simulink model "controller_stateflow_2021a"  (R2021a)
settings: Solver=FixedStepAuto  StartTime=0.0  StopTime=inf  FixedStep=0.05  RelTol=1e-3
PreLoadFcn:
  | rosinit();
model workspace (MAT data in the model file):
  SL_ROS_VariableLengthArrays_MaxSizes.CommonInfo.ArrayTruncateAction = 'EmitWarning'
  SL_ROS_VariableLengthArrays_MaxSizes.MsgTypeMap = containers.Map
  SL_ROS_VariableLengthArrays_MaxSizes.MsgTypeMap.serialization.keys = {'gazebo_msgs/LinkStates', 'trajectory_msgs/JointTrajectory', 'trajectory_msgs/JointTrajectoryPoint'}
  SL_ROS_VariableLengthArrays_MaxSizes.MsgTypeMap.serialization.values{1}(1).PropertyName = 'Name'
  SL_ROS_VariableLengthArrays_MaxSizes.MsgTypeMap.serialization.values{1}(1).DataType = 'std_msgs/String'
  SL_ROS_VariableLengthArrays_MaxSizes.MsgTypeMap.serialization.values{1}(1).MaxLength = 100
  SL_ROS_VariableLengthArrays_MaxSizes.MsgTypeMap.serialization.values{1}(2).PropertyName = 'Pose'
  SL_ROS_VariableLengthArrays_MaxSizes.MsgTypeMap.serialization.values{1}(2).DataType = 'geometry_msgs/Pose'
  SL_ROS_VariableLengthArrays_MaxSizes.MsgTypeMap.serialization.values{1}(2).MaxLength = 100
  SL_ROS_VariableLengthArrays_MaxSizes.MsgTypeMap.serialization.values{1}(3).PropertyName = 'Twist'
  SL_ROS_VariableLengthArrays_MaxSizes.MsgTypeMap.serialization.values{1}(3).DataType = 'geometry_msgs/Twist'
  SL_ROS_VariableLengthArrays_MaxSizes.MsgTypeMap.serialization.values{1}(3).MaxLength = 100
  SL_ROS_VariableLengthArrays_MaxSizes.MsgTypeMap.serialization.values{2}(1).PropertyName = 'JointNames'
  SL_ROS_VariableLengthArrays_MaxSizes.MsgTypeMap.serialization.values{2}(1).DataType = 'std_msgs/String'
  SL_ROS_VariableLengthArrays_MaxSizes.MsgTypeMap.serialization.values{2}(1).MaxLength = 16
  SL_ROS_VariableLengthArrays_MaxSizes.MsgTypeMap.serialization.values{2}(2).PropertyName = 'Points'
  SL_ROS_VariableLengthArrays_MaxSizes.MsgTypeMap.serialization.values{2}(2).DataType = 'trajectory_msgs/JointTrajectoryPoint'
  SL_ROS_VariableLengthArrays_MaxSizes.MsgTypeMap.serialization.values{2}(2).MaxLength = 1
  SL_ROS_VariableLengthArrays_MaxSizes.MsgTypeMap.serialization.values{3}(1).PropertyName = 'Accelerations'
  SL_ROS_VariableLengthArrays_MaxSizes.MsgTypeMap.serialization.values{3}(1).DataType = 'double'
  SL_ROS_VariableLengthArrays_MaxSizes.MsgTypeMap.serialization.values{3}(1).MaxLength = 128
  SL_ROS_VariableLengthArrays_MaxSizes.MsgTypeMap.serialization.values{3}(2).PropertyName = 'Effort'
  SL_ROS_VariableLengthArrays_MaxSizes.MsgTypeMap.serialization.values{3}(2).DataType = 'double'
  SL_ROS_VariableLengthArrays_MaxSizes.MsgTypeMap.serialization.values{3}(2).MaxLength = 128
  SL_ROS_VariableLengthArrays_MaxSizes.MsgTypeMap.serialization.values{3}(3).PropertyName = 'Positions'
  SL_ROS_VariableLengthArrays_MaxSizes.MsgTypeMap.serialization.values{3}(3).DataType = 'double'
  SL_ROS_VariableLengthArrays_MaxSizes.MsgTypeMap.serialization.values{3}(3).MaxLength = 7
  SL_ROS_VariableLengthArrays_MaxSizes.MsgTypeMap.serialization.values{3}(4).PropertyName = 'Velocities'
  SL_ROS_VariableLengthArrays_MaxSizes.MsgTypeMap.serialization.values{3}(4).DataType = 'double'
  SL_ROS_VariableLengthArrays_MaxSizes.MsgTypeMap.serialization.values{3}(4).MaxLength = 128
  SL_ROS_VariableLengthArrays_MaxSizes.MsgTypeMap.serialization.uniformity = 0
  SL_ROS_VariableLengthArrays_MaxSizes.MsgTypeMap.serialization.keyType = 'char'
  SL_ROS_VariableLengthArrays_MaxSizes.MsgTypeMap.serialization.valueType = 'any'
  pitch = -10
  restart = 0
values from neighbouring files (symbols this model uses):
  Pose = distance*inv(toPandatf)*Pose_d0    [inverseContoller3.m]    (also in inverseContoller4.m = distance*inv(toUR10etf)*Point_d0; inverseContoller_dual.m = inv(toUR10etf)*Point_d0; inverseContoller_dual2.m = inv(toUR10etf)*Point_d0)
undefined symbols (not defined in the file or in its folder): StartTime
libraries: robotlib x19, robotmaniplib x5, robotcorelib x3, robotgazebolib x1
(part 1 of 2)
settings Model: Creator=marco  LastModifiedBy=marco
settings OptimizationCC: EnhancedBackFolding=on  PassReuseOutputArgsAs=Individual arguments  ZeroExternalMemoryAtStartup=off  ZeroInternalMemoryAtStartup=off  MaxStackSize=64  OptimizeBlockOrder=speed  DifferentSizesBufferReuse=on  OptimizationCustomize=off  EfficientTunableParamExpr=on
settings DebuggingCC: ParameterTunabilityLossMsg=error  UnconnectedInputMsg=none  UnconnectedOutputMsg=none  UnconnectedLineMsg=none
settings HardwareCC: ProdBitPerPointer=32  ProdBitPerSizeT=32  ProdBitPerPtrDiffT=32  ProdLargestAtomicFloat=None  ProdIntDivRoundTo=Undefined  ProdEndianess=Unspecified  ProdWordSize=32  ProdHWDeviceType=Generic->Unspecified (assume 32-bit Generic)
settings ModelReferenceCC: EnableRefExpFcnMdlSchedulingChecks=off
settings SFSimCC: MATLABDynamicMemAlloc=off
settings RTWCC: SystemTargetFile=ert.tlc  HardwareBoard=Robot Operating System (ROS)  TLCOptions="-aInlineSetEventsForThisBaseRateFcn=TLC_FALSE -aSuppressMultiTaskScheduler=TLC_FALSE  -aRateBasedStepFcn=0"  TemplateMakefile=ert_default_tmf  Toolchain=Catkin  TargetLang=C++  DLArmComputeVersion=20.02.1
settings CodeAppCC: ForceParamTrailComments=on  IgnoreCustomStorageClasses=off  OperatorAnnotations=on  SimulinkDataObjDesc=on  SFDataObjDesc=on  InsertBlockDesc=on

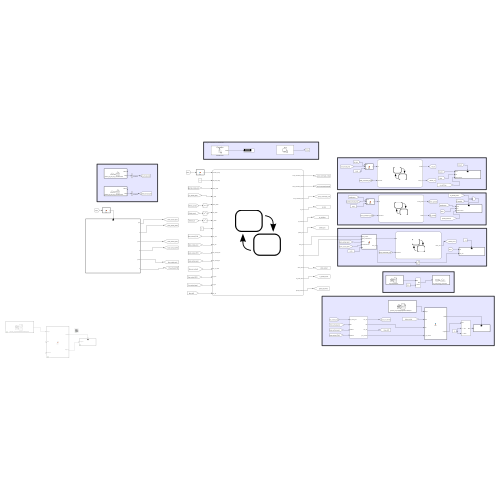
[thumbnail: Simulink's stored preview of the top-level diagram]
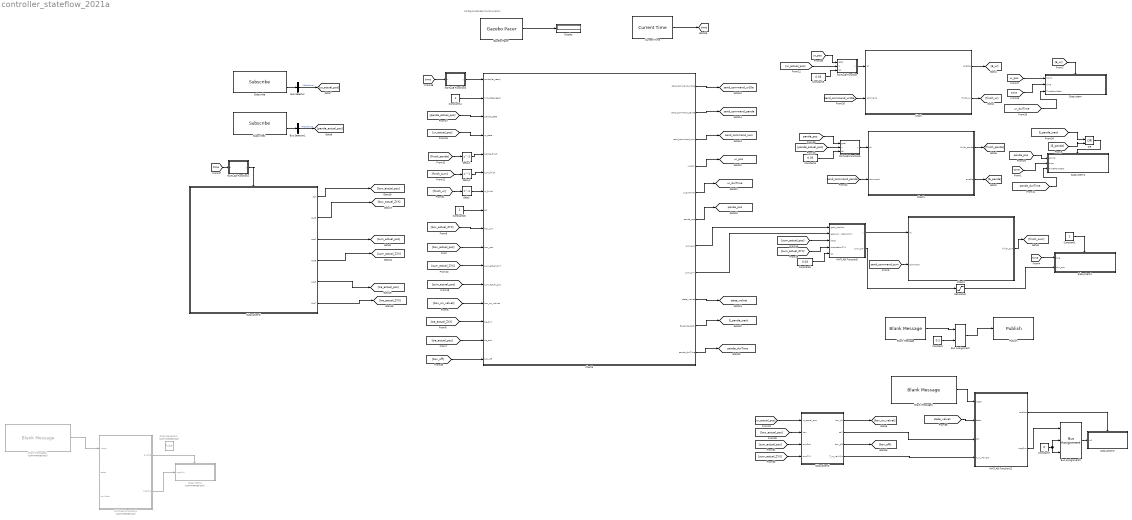
== system controller_stateflow_2021a ==
  note: Configure Gazebo Co-Simulation
  Blank Message : robotlib/Blank Message  messageClass=Message  entityType=std_msgs/Float64  messageType=std_msgs/Float64  SampleTime=inf  legacyBusStruct=off
  Blank Message1 : robotlib/Blank Message  messageClass=Service Request  entityType=gazebo_msgs/ApplyBodyWrench  messageType=gazebo_msgs/ApplyBodyWrenchRequest  SampleTime=-1  legacyBusStruct=off
  Blank Message2 : robotlib/Blank Message  Commented=on  messageClass=Service Request  entityType=gazebo_msgs/SetModelState  messageType=gazebo_msgs/SetModelStateRequest  SampleTime=-1  legacyBusStruct=off
  Bus Assignment : BusAssignment  AssignedSignals=Data
  Bus Assignment2 : BusAssignment  AssignedSignals=StartTime.Sec,StartTime.Nsec
  Bus Selector : BusSelector  OutputSignals=Actual.Positions
  Bus Selector1 : BusSelector  OutputSignals=Actual.Positions
  Chart : Stateflow chart  TreatAsAtomicUnit=on
  Chart1 : Stateflow chart  TreatAsAtomicUnit=on
  Chart2 : Stateflow chart  TreatAsAtomicUnit=on
  Chart3 : Stateflow chart  TreatAsAtomicUnit=on
  Constant : Constant  Value=0.2
  Constant1 : Constant
  Constant11 : Constant
  Constant20 : Constant
  Constant3 : Constant  Value=0.03
  Constant4 : Constant  Value=0.03
  Constant6 : Constant  Value=0.03
  Constant7 : Constant  Value=0
  Current Time : robotlib/Current Time  OutputFormat=bus  SampleTime=-1  ModelName=controller_stateflow
  Delay : Delay  DelayLength=1  InitialCondition=0
  Delay1 : Delay  DelayLength=1  InitialCondition=0
  Delay2 : Delay  DelayLength=1  InitialCondition=0
  Display : Display
  Gazebo Pacer : robotgazebolib/Gazebo Pacer  ResetBehavior=Reset Gazebo simulation time  SampleTime=0.05
  MATLAB Function : MATLAB Function  TreatAsAtomicUnit=on
  MATLAB Function1 : MATLAB Function  TreatAsAtomicUnit=on
  MATLAB Function12 : MATLAB Function  TreatAsAtomicUnit=on
  MATLAB Function14 : MATLAB Function  Commented=on  TreatAsAtomicUnit=on
  MATLAB Function2 : MATLAB Function  TreatAsAtomicUnit=on
  MATLAB Function3 : MATLAB Function  TreatAsAtomicUnit=on
  MATLAB Function5 : MATLAB Function  TreatAsAtomicUnit=on
  OR : Logic  Operator=OR  IconShape=distinctive  AllPortsSameDT=off  OutDataTypeStr=boolean
  Publish : robotlib/Publish  topicSource=Select from ROS network  topic=/right_hand_v1s/synergy_command  messageType=std_msgs/Float64  legacyBusStruct=off  messageQueueLength=1
  Pulse Generator : DiscretePulseGenerator  Commented=on  PulseType=Time based  Period=10  PulseWidth=0.1
  Saturation : Saturate  UpperLimit=0.2  LowerLimit=-0.2
  Subscribe : robotlib/Subscribe  topicSource=Select from ROS network  topic=/ur10e_eff_joint_traj_controller/state  messageType=control_msgs/JointTrajectoryControllerState  SampleTime=-1  legacyBusStruct=off  messageQueueLength=1
  Subscribe1 : robotlib/Subscribe  topicSource=Select from ROS network  topic=/panda_eff_joint_traj_controller/state  messageType=control_msgs/JointTrajectoryControllerState  SampleTime=-1  legacyBusStruct=off  messageQueueLength=1
  Subsystem : Subsystem
  Subsystem1 : Subsystem
  Subsystem2 : Subsystem
  Subsystem3 : Subsystem
  Subsystem4 : Subsystem  Commented=on
  Subsystem5 : Subsystem
  Subsystem6 : Subsystem
  tag scope: E_panda_track=global, panda_durTime=global, panda_pos=global, send_command_panda=global, send_command_sum=global, send_command_ur10e=global, state_velvet=global, time=global, ur_durTime=global, ur_pos=global
  wires:
  [time] -> Subsystem1/2(time)
  [E_ur] -> Subsystem/Enable
  Chart/1(enable) -> [E_ur]
  Subscribe/2 -> Bus Selector/1
  Constant3/1 -> MATLAB Function/3(tol)
  MATLAB Function/1(y) -> Chart/1(ok)
  MATLAB Function3/1(y) -> Chart1/1(ok)
  Constant4/1 -> MATLAB Function3/3(tol)
  Subscribe1/2 -> Bus Selector1/1
  Chart1/2(enable) -> [E_panda]
  [E_panda] -> OR/2
  [panda_pos] -> Subsystem1/1(points)
  Constant6/1 -> MATLAB Function5/5(tol)
  MATLAB Function5/1(y) -> Chart2/1(ok)
  MATLAB Function5/2(sum_cntr) -> Saturation/1
  Constant1/1 -> Subsystem2/Enable
  Chart/2(finish_ur) -> [finish_ur]
  Chart1/1(finish_panda) -> [finish_panda]
  Saturation/1 -> Subsystem2/2(sum_cntr)
  MATLAB Function1/1(y) -> Subsystem6/Enable
  Constant11/1 -> Chart3/2(link_state_ready)
  Bus Selector/1 -> [ur_actual_pos]  "<Positions>"
  Bus Selector1/1 -> [panda_actual_pos]  "<Positions>"
  [ur_actual_pos] -> MATLAB Function/2(u)
  [sum_actual_ZYX] -> MATLAB Function5/4(orientationZYX)
  [panda_actual_pos] -> MATLAB Function3/2(u)
  [panda_actual_pos] -> Chart3/3(panda_state)
  [ur_actual_pos] -> Chart3/4(ur_state)
  [finish_sum] -> Delay2/1
  [finish_ur] -> Delay/1
  Chart3/7(sum_pos) -> MATLAB Function5/1(goal_position)
  Delay/1 -> Chart3/7(ur_finish)
  Constant20/1 -> Chart3/8(go)
  [time] -> Subsystem/2(time)
  Chart3/1(send_command_ur10e) -> [send_command_ur10e]
  [send_command_ur10e] -> Chart/2(command)
  [ur_pos] -> Subsystem/1(Point)
  [ur_pos] -> MATLAB Function/1(goal)
  Chart3/3(send_command_sum) -> [send_command_sum]
  Chart3/2(send_command_panda) -> [send_command_panda]
  Chart3/4(ur_pos) -> [ur_pos]
  Chart3/6(panda_pos) -> [panda_pos]
  [send_command_panda] -> Chart1/2(command)
  [panda_pos] -> MATLAB Function3/1(goal)
  [finish_panda] -> Delay1/1
  Delay1/1 -> Chart3/5(panda_finish)
  [time] -> Subsystem2/1(time)
  [send_command_sum] -> Chart2/2(command)
  Chart2/1(finish_sum) -> [finish_sum]
  Delay2/1 -> Chart3/6(sum_finish)
  [box_actual_ZYX] -> Chart3/9(box_ZYX)
  Chart3/8(sum_ZYX) -> MATLAB Function5/2(goal_orientationZYX)
  [box_actual_pos] -> Chart3/10(box_pos)
  [sum_actual_pos] -> MATLAB Function5/3(pose)
  [sum_actual_ZYX] -> Chart3/11(sum_actual_ZYX)
  [sum_actual_pos] -> Chart3/12(sum_actual_pos)
  [box_on_velvet] -> Chart3/13(box_on_velvet)
  Bus Assignment/1 -> Publish/1
  Blank Message/1 -> Bus Assignment/1
  Constant/1 -> Bus Assignment/2
  [tra_actual_pos] -> Chart3/15(tra_pos)
  [tra_actual_ZYX] -> Chart3/14(tra_ZYX)
  OR/1 -> Subsystem1/Enable
  [panda_durTime] -> Subsystem1/3(TimeFromStart)
  Chart3/5(ur_durTime) -> [ur_durTime]
  [ur_durTime] -> Subsystem/3(TimeFromStart)
  Chart3/11(panda_durTime) -> [panda_durTime]
  MATLAB Function12/1(enable) -> Subsystem3/Enable
  Blank Message1/1 -> MATLAB Function12/1(msgIn)
  Bus Assignment2/1 -> Subsystem3/1(In1)
  Constant7/1 -> Bus Assignment2/3, Bus Assignment2/2
  MATLAB Function12/2(msgOut) -> Bus Assignment2/1
  Chart3/10(E_panda_track) -> [E_panda_track]
  [E_panda_track] -> OR/1
  Blank Message2/1 -> MATLAB Function14/1(msgIn)
  MATLAB Function14/2(msgOut) -> Subsystem4/1(msgOut)
  MATLAB Function14/1(enable) -> Subsystem4/Enable
  [box_off] -> Chart3/16(box_off)
  Chart3/9(state_velvet) -> [state_velvet]
  [state_velvet] -> MATLAB Function12/2(state)
  [ur_actual_pos] -> Subsystem5/1(ur_actual_pos)
  [box_actual_pos] -> Subsystem5/2(box)
  [sum_actual_pos] -> Subsystem5/3(sumPos)
  [sum_actual_ZYX] -> Subsystem5/4(sumZYX)
  Subsystem5/1(box_ok) -> [box_on_velvet]
  Subsystem5/2(coll) -> MATLAB Function12/3(coll)
  Subsystem5/3(box_off) -> [box_off]
  Subsystem5/4(T_ur_velvCnt) -> MATLAB Function12/4(T_ur_velvCnt)
  Gazebo Pacer/1 -> Display/1
  Subsystem6/1(pos) -> [box_actual_pos]
  Subsystem6/2(Out2) -> [box_actual_ZYX]
  Subsystem6/3(pos1) -> [sum_actual_pos]
  Subsystem6/4(Out5) -> [sum_actual_ZYX]
  Subsystem6/5(pos2) -> [tra_actual_pos]
  Subsystem6/6(Out7) -> [tra_actual_ZYX]
  [time] -> MATLAB Function1/1(u)
  Current Time/1 -> [time]
  [time] -> MATLAB Function2/1(u)
  MATLAB Function2/1(y) -> Chart3/1(controller_ready)

== system controller_stateflow_2021a/Chart3/THE_END ==
  go : Inport
  Action Port : ActionPort
      settings: CopyFcn=Stateflow.SLINSF.SimulinkMan.removeBlockPreDeleteFcn  PreDeleteFcn=Stateflow.SLINSF.SimulinkMan.unsafePredeleteFcn
  Stop Simulation : Stop
  wires:
  go/1 -> Stop Simulation/1

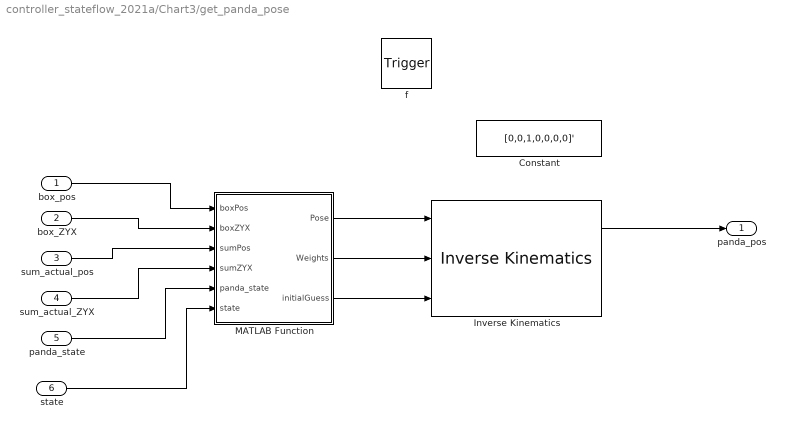
== system controller_stateflow_2021a/Chart3/get_panda_pose ==
  box_pos : Inport  OutDataTypeStr=double  PortDimensions=[3,1]
  box_ZYX : Inport  Port=2  OutDataTypeStr=double  PortDimensions=[3,1]
  sum_actual_pos : Inport  Port=3  OutDataTypeStr=double  PortDimensions=[3,1]
  sum_actual_ZYX : Inport  Port=4  OutDataTypeStr=double  PortDimensions=[3,1]
  panda_state : Inport  Port=5  OutDataTypeStr=double  PortDimensions=[7,1]
  state : Inport  Port=6  OutDataTypeStr=double  PortDimensions=1
  f : TriggerPort  TriggerType=function-call  VariantControl=(inherit)
      settings: CopyFcn=Stateflow.SLINSF.SimulinkMan.removeBlockPreDeleteFcn  PreDeleteFcn=Stateflow.SLINSF.SimulinkMan.unsafePredeleteFcn
  Constant : Constant  Value=[0,0,1,0,0,0,0]'
  Inverse Kinematics : robotmaniplib/Inverse Kinematics  RigidBodyTree=franka  EndEffector=hand_link  ShowInfo=on  SolverName=BFGS Gradient Projection  EnforceJointLimits=on  MaxIterations=1500  MaxTime=10  GradientTolerance=1e-7  SolutionTolerance=1e-6  StepTolerance=1e-14  ErrorChangeTolerance=1e-12  UseErrorDamping=on  DampingBias=0.0025  SimulateUsing=Interpreted execution
  MATLAB Function : MATLAB Function  TreatAsAtomicUnit=on
  panda_pos : Outport
  wires:
  panda_state/1 -> MATLAB Function/5(panda_state)
  box_pos/1 -> MATLAB Function/1(boxPos)
  box_ZYX/1 -> MATLAB Function/2(boxZYX)
  sum_actual_pos/1 -> MATLAB Function/3(sumPos)
  sum_actual_ZYX/1 -> MATLAB Function/4(sumZYX)
  MATLAB Function/1(Pose) -> Inverse Kinematics/1
  MATLAB Function/2(Weights) -> Inverse Kinematics/2
  MATLAB Function/3(initialGuess) -> Inverse Kinematics/3
  Inverse Kinematics/1 -> panda_pos/1
  state/1 -> MATLAB Function/6(state)

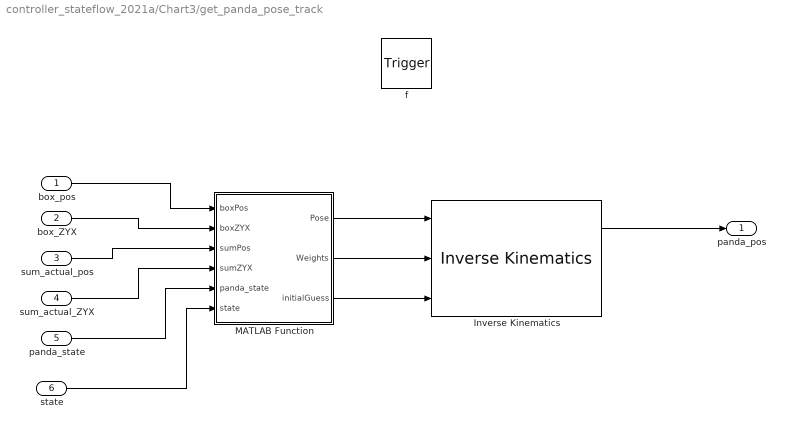
== system controller_stateflow_2021a/Chart3/get_panda_pose_track ==
  box_pos : Inport  OutDataTypeStr=double  PortDimensions=[3,1]
  box_ZYX : Inport  Port=2  OutDataTypeStr=double  PortDimensions=[3,1]
  sum_actual_pos : Inport  Port=3  OutDataTypeStr=double  PortDimensions=[3,1]
  sum_actual_ZYX : Inport  Port=4  OutDataTypeStr=double  PortDimensions=[3,1]
  panda_state : Inport  Port=5  OutDataTypeStr=double  PortDimensions=[7,1]
  state : Inport  Port=6  OutDataTypeStr=double  PortDimensions=1
  f : TriggerPort  TriggerType=function-call  VariantControl=(inherit)
      settings: CopyFcn=Stateflow.SLINSF.SimulinkMan.removeBlockPreDeleteFcn  PreDeleteFcn=Stateflow.SLINSF.SimulinkMan.unsafePredeleteFcn
  Inverse Kinematics : robotmaniplib/Inverse Kinematics  RigidBodyTree=franka  EndEffector=hand_link  ShowInfo=on  SolverName=BFGS Gradient Projection  EnforceJointLimits=on  MaxIterations=1500  MaxTime=10  GradientTolerance=1e-7  SolutionTolerance=1e-6  StepTolerance=1e-14  ErrorChangeTolerance=1e-12  UseErrorDamping=on  DampingBias=0.0025  SimulateUsing=Interpreted execution
  MATLAB Function : MATLAB Function  TreatAsAtomicUnit=on
  panda_pos : Outport
  wires:
  panda_state/1 -> MATLAB Function/5(panda_state)
  box_pos/1 -> MATLAB Function/1(boxPos)
  box_ZYX/1 -> MATLAB Function/2(boxZYX)
  sum_actual_pos/1 -> MATLAB Function/3(sumPos)
  sum_actual_ZYX/1 -> MATLAB Function/4(sumZYX)
  MATLAB Function/1(Pose) -> Inverse Kinematics/1
  MATLAB Function/2(Weights) -> Inverse Kinematics/2
  MATLAB Function/3(initialGuess) -> Inverse Kinematics/3
  Inverse Kinematics/1 -> panda_pos/1
  state/1 -> MATLAB Function/6(state)

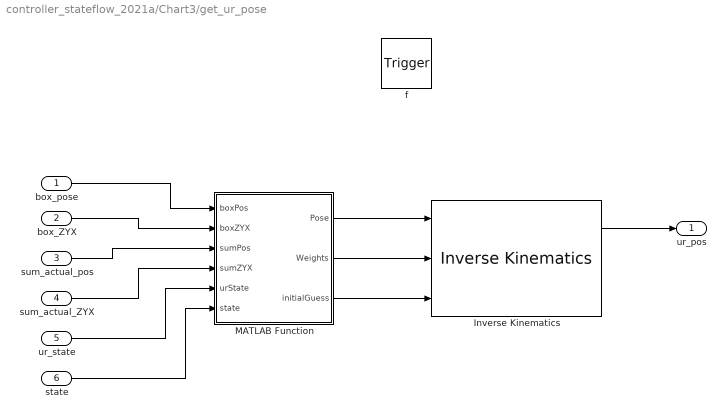
== system controller_stateflow_2021a/Chart3/get_ur_pose ==
  box_pose : Inport  OutDataTypeStr=double  PortDimensions=[3,1]
  box_ZYX : Inport  Port=2  OutDataTypeStr=double  PortDimensions=[3,1]
  sum_actual_pos : Inport  Port=3  OutDataTypeStr=double  PortDimensions=[3,1]
  sum_actual_ZYX : Inport  Port=4  OutDataTypeStr=double  PortDimensions=[3,1]
  ur_state : Inport  Port=5  OutDataTypeStr=double  PortDimensions=[7,1]
  state : Inport  Port=6  OutDataTypeStr=double  PortDimensions=1
  f : TriggerPort  TriggerType=function-call  VariantControl=(inherit)
      settings: CopyFcn=Stateflow.SLINSF.SimulinkMan.removeBlockPreDeleteFcn  PreDeleteFcn=Stateflow.SLINSF.SimulinkMan.unsafePredeleteFcn
  Inverse Kinematics : robotmaniplib/Inverse Kinematics  RigidBodyTree=ur10e  EndEffector=ee_link  ShowInfo=on  SolverName=BFGS Gradient Projection  EnforceJointLimits=on  MaxIterations=1500  MaxTime=10  GradientTolerance=1e-7  SolutionTolerance=1e-6  StepTolerance=1e-14  ErrorChangeTolerance=1e-12  UseErrorDamping=on  DampingBias=0.0025  SimulateUsing=Interpreted execution
  MATLAB Function : MATLAB Function  TreatAsAtomicUnit=on
  ur_pos : Outport
  wires:
  ur_state/1 -> MATLAB Function/5(urState)
  Inverse Kinematics/1 -> ur_pos/1
  box_pose/1 -> MATLAB Function/1(boxPos)
  box_ZYX/1 -> MATLAB Function/2(boxZYX)
  sum_actual_pos/1 -> MATLAB Function/3(sumPos)
  sum_actual_ZYX/1 -> MATLAB Function/4(sumZYX)
  MATLAB Function/1(Pose) -> Inverse Kinematics/1
  MATLAB Function/2(Weights) -> Inverse Kinematics/2
  MATLAB Function/3(initialGuess) -> Inverse Kinematics/3
  state/1 -> MATLAB Function/6(state)

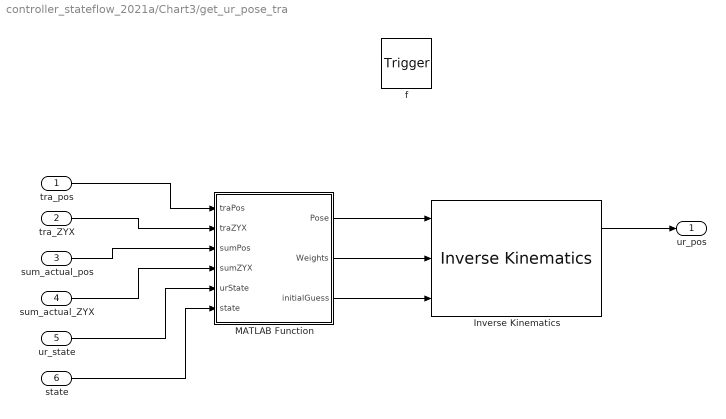
== system controller_stateflow_2021a/Chart3/get_ur_pose_tra ==
  tra_pos : Inport  OutDataTypeStr=double  PortDimensions=[3,1]
  tra_ZYX : Inport  Port=2  OutDataTypeStr=double  PortDimensions=[3,1]
  sum_actual_pos : Inport  Port=3  OutDataTypeStr=double  PortDimensions=[3,1]
  sum_actual_ZYX : Inport  Port=4  OutDataTypeStr=double  PortDimensions=[3,1]
  ur_state : Inport  Port=5  OutDataTypeStr=double  PortDimensions=[7,1]
  state : Inport  Port=6  OutDataTypeStr=double  PortDimensions=1
  f : TriggerPort  TriggerType=function-call  VariantControl=(inherit)
      settings: CopyFcn=Stateflow.SLINSF.SimulinkMan.removeBlockPreDeleteFcn  PreDeleteFcn=Stateflow.SLINSF.SimulinkMan.unsafePredeleteFcn
  Inverse Kinematics : robotmaniplib/Inverse Kinematics  RigidBodyTree=ur10e  EndEffector=ee_link  ShowInfo=on  SolverName=BFGS Gradient Projection  EnforceJointLimits=on  MaxIterations=1500  MaxTime=10  GradientTolerance=1e-7  SolutionTolerance=1e-6  StepTolerance=1e-14  ErrorChangeTolerance=1e-12  UseErrorDamping=on  DampingBias=0.0025  SimulateUsing=Interpreted execution
  MATLAB Function : MATLAB Function  TreatAsAtomicUnit=on
  ur_pos : Outport
  wires:
  ur_state/1 -> MATLAB Function/5(urState)
  Inverse Kinematics/1 -> ur_pos/1
  tra_pos/1 -> MATLAB Function/1(traPos)
  tra_ZYX/1 -> MATLAB Function/2(traZYX)
  sum_actual_pos/1 -> MATLAB Function/3(sumPos)
  sum_actual_ZYX/1 -> MATLAB Function/4(sumZYX)
  MATLAB Function/1(Pose) -> Inverse Kinematics/1
  MATLAB Function/2(Weights) -> Inverse Kinematics/2
  MATLAB Function/3(initialGuess) -> Inverse Kinematics/3
  state/1 -> MATLAB Function/6(state)

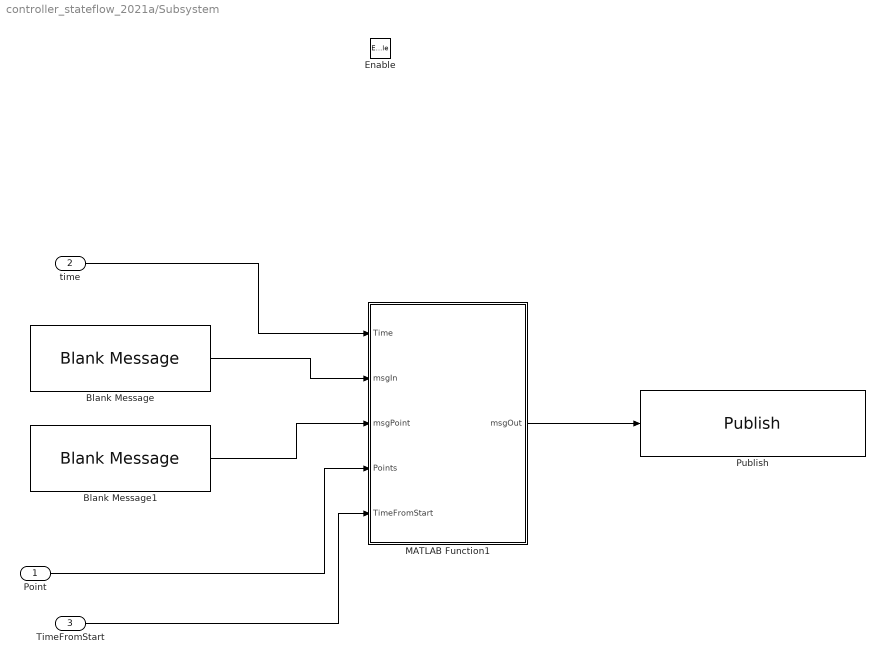
== system controller_stateflow_2021a/Subsystem ==
  Point : Inport
  time : Inport  Port=2
  TimeFromStart : Inport  Port=3
  Enable : EnablePort
  Blank Message : robotlib/Blank Message  messageClass=Message  entityType=trajectory_msgs/JointTrajectory  messageType=trajectory_msgs/JointTrajectory  SampleTime=inf  legacyBusStruct=off
  Blank Message1 : robotlib/Blank Message  messageClass=Message  entityType=trajectory_msgs/JointTrajectoryPoint  messageType=trajectory_msgs/JointTrajectoryPoint  SampleTime=inf  legacyBusStruct=off
  MATLAB Function1 : MATLAB Function  TreatAsAtomicUnit=on
  Publish : robotlib/Publish  topicSource=Select from ROS network  topic=/ur10e_eff_joint_traj_controller/command  messageType=trajectory_msgs/JointTrajectory  legacyBusStruct=off  messageQueueLength=1
  wires:
  Blank Message/1 -> MATLAB Function1/2(msgIn)
  Blank Message1/1 -> MATLAB Function1/3(msgPoint)
  MATLAB Function1/1(msgOut) -> Publish/1
  Point/1 -> MATLAB Function1/4(Points)
  time/1 -> MATLAB Function1/1(Time)
  TimeFromStart/1 -> MATLAB Function1/5(TimeFromStart)

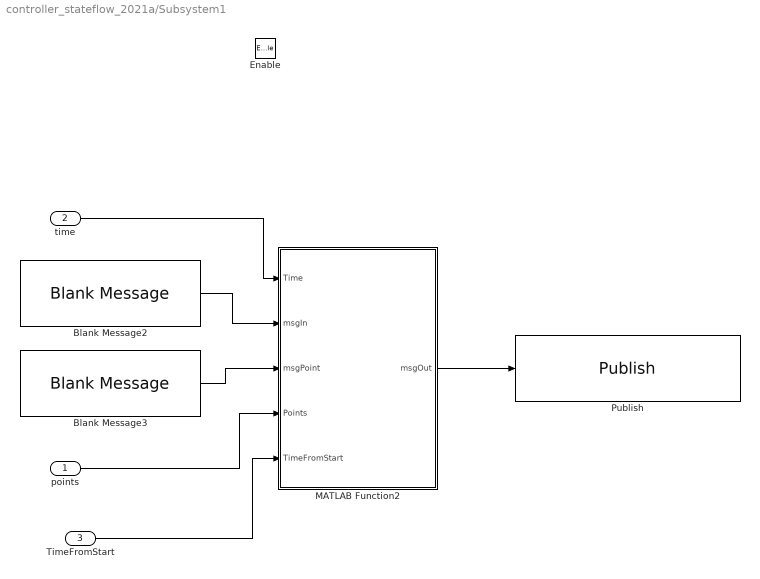
== system controller_stateflow_2021a/Subsystem1 ==
  points : Inport
  time : Inport  Port=2
  TimeFromStart : Inport  Port=3
  Enable : EnablePort
  Blank Message2 : robotlib/Blank Message  messageClass=Message  entityType=trajectory_msgs/JointTrajectory  messageType=trajectory_msgs/JointTrajectory  SampleTime=inf  legacyBusStruct=off
  Blank Message3 : robotlib/Blank Message  messageClass=Message  entityType=trajectory_msgs/JointTrajectoryPoint  messageType=trajectory_msgs/JointTrajectoryPoint  SampleTime=inf  legacyBusStruct=off
  MATLAB Function2 : MATLAB Function  TreatAsAtomicUnit=on
  Publish : robotlib/Publish  topicSource=Select from ROS network  topic=/panda_eff_joint_traj_controller/command  messageType=trajectory_msgs/JointTrajectory  legacyBusStruct=off  messageQueueLength=1
  wires:
  time/1 -> MATLAB Function2/1(Time)
  Blank Message3/1 -> MATLAB Function2/3(msgPoint)
  Blank Message2/1 -> MATLAB Function2/2(msgIn)
  MATLAB Function2/1(msgOut) -> Publish/1
  points/1 -> MATLAB Function2/4(Points)
  TimeFromStart/1 -> MATLAB Function2/5(TimeFromStart)

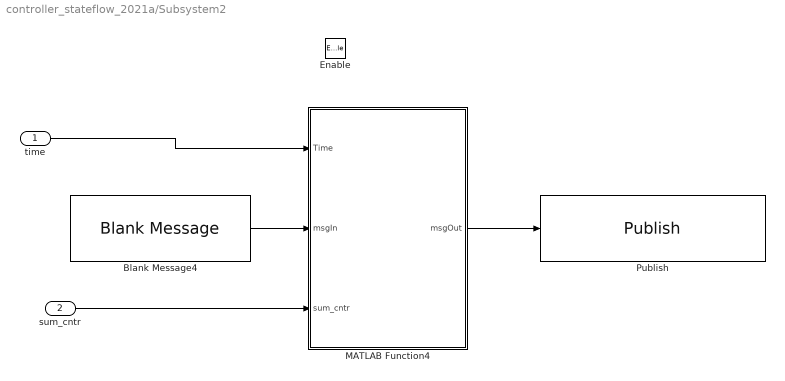
== system controller_stateflow_2021a/Subsystem2 ==
  time : Inport
  sum_cntr : Inport  Port=2
  Enable : EnablePort
  Blank Message4 : robotlib/Blank Message  messageClass=Message  entityType=geometry_msgs/Twist  messageType=geometry_msgs/Twist  SampleTime=inf  legacyBusStruct=off
  MATLAB Function4 : MATLAB Function  TreatAsAtomicUnit=on
  Publish : robotlib/Publish  topicSource=Select from ROS network  topic=/robotnik_base_control/cmd_vel  messageType=geometry_msgs/Twist  legacyBusStruct=off  messageQueueLength=1
  wires:
  Blank Message4/1 -> MATLAB Function4/2(msgIn)
  MATLAB Function4/1(msgOut) -> Publish/1
  time/1 -> MATLAB Function4/1(Time)
  sum_cntr/1 -> MATLAB Function4/3(sum_cntr)

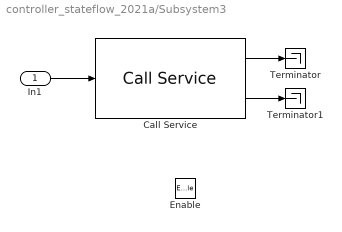
== system controller_stateflow_2021a/Subsystem3 ==
  In1 : Inport
  Enable : EnablePort
  Call Service : robotlib/Call Service  topicSource=Select from ROS network  service=/gazebo/apply_body_wrench  serviceType=gazebo_msgs/ApplyBodyWrench  connectionTimeout=5  keepPersistent=off  ShowErrorCodeOutput=on  legacyBusStruct=off
  Terminator : Terminator
  Terminator1 : Terminator
  wires:
  Call Service/1 -> Terminator/1
  Call Service/2 -> Terminator1/1
  In1/1 -> Call Service/1

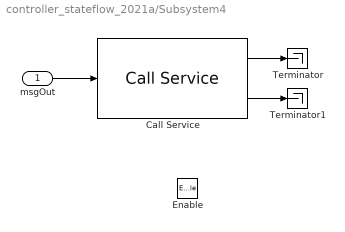
== system controller_stateflow_2021a/Subsystem4 ==
  msgOut : Inport
  Enable : EnablePort
  Call Service : robotlib/Call Service  topicSource=Select from ROS network  service=/gazebo/set_model_state  serviceType=gazebo_msgs/SetModelState  connectionTimeout=5  keepPersistent=off  ShowErrorCodeOutput=on  legacyBusStruct=off
  Terminator : Terminator
  Terminator1 : Terminator
  wires:
  msgOut/1 -> Call Service/1
  Call Service/2 -> Terminator1/1
  Call Service/1 -> Terminator/1

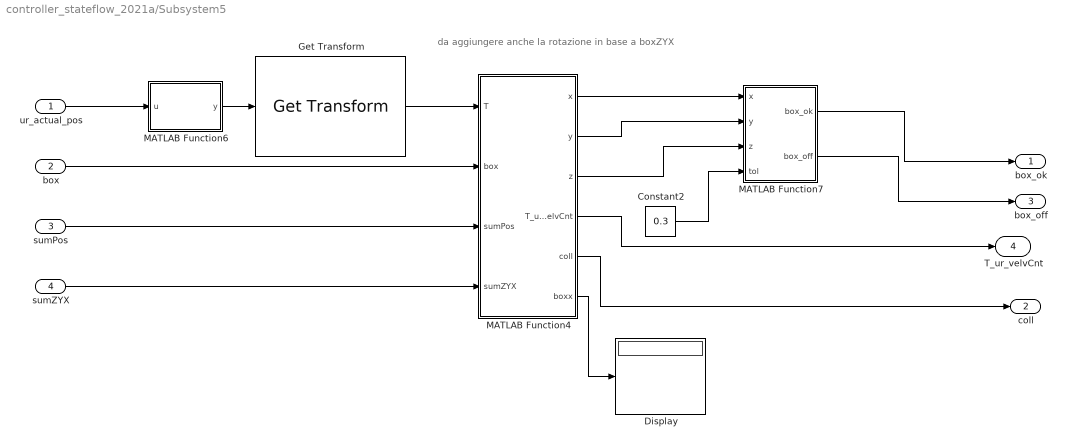
== system controller_stateflow_2021a/Subsystem5 ==
  note: da aggiungere anche la rotazione in base a boxZYX
  ur_actual_pos : Inport
  box : Inport  Port=2
  sumPos : Inport  Port=3
  sumZYX : Inport  Port=4
  Constant2 : Constant  Value=0.3
  Display : Display
  Get Transform : robotmaniplib/Get Transform  RigidBodyTree=ur10e  SourceBody=tool0  TargetBody=world  SimulateUsing=Interpreted execution
  MATLAB Function4 : MATLAB Function  TreatAsAtomicUnit=on
  MATLAB Function6 : MATLAB Function  TreatAsAtomicUnit=on
  MATLAB Function7 : MATLAB Function  TreatAsAtomicUnit=on
  box_ok : Outport
  coll : Outport  Port=2
  box_off : Outport  Port=3
  T_ur_velvCnt : Outport  Port=4
  wires:
  MATLAB Function7/1(box_ok) -> box_ok/1
  Get Transform/1 -> MATLAB Function4/1(T)
  MATLAB Function4/1(x) -> MATLAB Function7/1(x)
  Constant2/1 -> MATLAB Function7/4(tol)
  MATLAB Function7/2(box_off) -> box_off/1
  MATLAB Function4/3(z) -> MATLAB Function7/3(z)
  MATLAB Function6/1(y) -> Get Transform/1
  MATLAB Function4/2(y) -> MATLAB Function7/2(y)
  MATLAB Function4/5(coll) -> coll/1
  box/1 -> MATLAB Function4/2(box)
  ur_actual_pos/1 -> MATLAB Function6/1(u)
  sumPos/1 -> MATLAB Function4/3(sumPos)
  MATLAB Function4/4(T_ur_velvCnt) -> T_ur_velvCnt/1
  sumZYX/1 -> MATLAB Function4/4(sumZYX)
  MATLAB Function4/6(boxx) -> Display/1

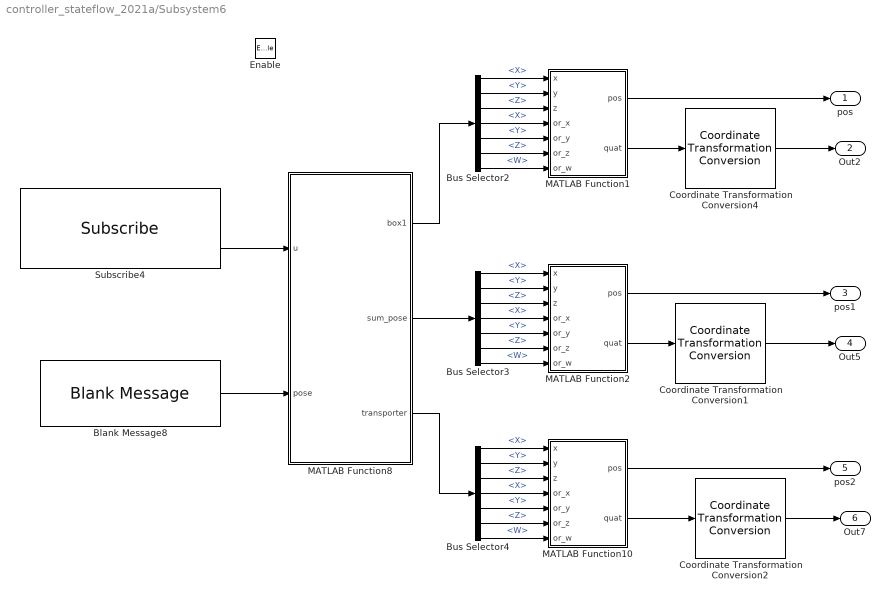
== system controller_stateflow_2021a/Subsystem6 ==
  Enable : EnablePort
  Blank Message8 : robotlib/Blank Message  messageClass=Message  entityType=geometry_msgs/Pose  messageType=geometry_msgs/Pose  SampleTime=inf  legacyBusStruct=off
  Bus Selector2 : BusSelector  OutputSignals=Position.X,Position.Y,Position.Z,Orientation.X,Orientation.Y,Orientation.Z,Orientation.W
  Bus Selector3 : BusSelector  OutputSignals=Position.X,Position.Y,Position.Z,Orientation.X,Orientation.Y,Orientation.Z,Orientation.W
  Bus Selector4 : BusSelector  OutputSignals=Position.X,Position.Y,Position.Z,Orientation.X,Orientation.Y,Orientation.Z,Orientation.W
  Coordinate Transformation Conversion1 : robotcorelib/Coordinate Transformation Conversion  InputRepresentation=Quaternion  InputEulerSequence=ZYX  ShowTrVecInputPort=on  OutputRepresentation=Euler Angles  OutputEulerSequence=ZYX  ShowTrVecOutputPort=on  SimulateUsing=Interpreted execution
  Coordinate Transformation Conversion2 : robotcorelib/Coordinate Transformation Conversion  InputRepresentation=Quaternion  InputEulerSequence=ZYX  ShowTrVecInputPort=on  OutputRepresentation=Euler Angles  OutputEulerSequence=ZYX  ShowTrVecOutputPort=on  SimulateUsing=Interpreted execution
  Coordinate Transformation Conversion4 : robotcorelib/Coordinate Transformation Conversion  InputRepresentation=Quaternion  InputEulerSequence=ZYX  ShowTrVecInputPort=on  OutputRepresentation=Euler Angles  OutputEulerSequence=ZYX  ShowTrVecOutputPort=on  SimulateUsing=Interpreted execution
  MATLAB Function1 : MATLAB Function  TreatAsAtomicUnit=on
  MATLAB Function10 : MATLAB Function  TreatAsAtomicUnit=on
  MATLAB Function2 : MATLAB Function  TreatAsAtomicUnit=on
  MATLAB Function8 : MATLAB Function  TreatAsAtomicUnit=on
  Subscribe4 : robotlib/Subscribe  topicSource=Select from ROS network  topic=/gazebo/link_states  messageType=gazebo_msgs/LinkStates  SampleTime=-1  legacyBusStruct=off  messageQueueLength=1
  pos : Outport
  Out2 : Outport  Port=2
  pos1 : Outport  Port=3
  Out5 : Outport  Port=4
  pos2 : Outport  Port=5
  Out7 : Outport  Port=6
  wires:
  Bus Selector2/7 -> MATLAB Function1/7(or_w)  "<W>"
  Bus Selector4/6 -> MATLAB Function10/6(or_z)  "<Z>"
  Bus Selector2/2 -> MATLAB Function1/2(y)  "<Y>"
  Subscribe4/2 -> MATLAB Function8/1(u)
  MATLAB Function1/1(pos) -> pos/1
  Bus Selector4/5 -> MATLAB Function10/5(or_y)  "<Y>"
  Coordinate Transformation Conversion2/1 -> Out7/1
  MATLAB Function10/1(pos) -> pos2/1
  MATLAB Function8/1(box1) -> Bus Selector2/1
  Coordinate Transformation Conversion4/1 -> Out2/1
  Bus Selector2/6 -> MATLAB Function1/6(or_z)  "<Z>"
  Bus Selector2/5 -> MATLAB Function1/5(or_y)  "<Y>"
  MATLAB Function10/2(quat) -> Coordinate Transformation Conversion2/1
  Bus Selector3/1 -> MATLAB Function2/1(x)  "<X>"
  Bus Selector4/1 -> MATLAB Function10/1(x)  "<X>"
  Bus Selector3/5 -> MATLAB Function2/5(or_y)  "<Y>"
  Blank Message8/1 -> MATLAB Function8/2(pose)
  MATLAB Function2/1(pos) -> pos1/1
  Bus Selector4/4 -> MATLAB Function10/4(or_x)  "<X>"
  Bus Selector3/3 -> MATLAB Function2/3(z)  "<Z>"
  Bus Selector4/2 -> MATLAB Function10/2(y)  "<Y>"
  Coordinate Transformation Conversion1/1 -> Out5/1
  MATLAB Function2/2(quat) -> Coordinate Transformation Conversion1/1
  MATLAB Function8/2(sum_pose) -> Bus Selector3/1
  Bus Selector3/6 -> MATLAB Function2/6(or_z)  "<Z>"
  Bus Selector4/3 -> MATLAB Function10/3(z)  "<Z>"
  Bus Selector2/1 -> MATLAB Function1/1(x)  "<X>"
  Bus Selector3/4 -> MATLAB Function2/4(or_x)  "<X>"
  Bus Selector3/2 -> MATLAB Function2/2(y)  "<Y>"
  MATLAB Function1/2(quat) -> Coordinate Transformation Conversion4/1
  Bus Selector2/3 -> MATLAB Function1/3(z)  "<Z>"
  Bus Selector4/7 -> MATLAB Function10/7(or_w)  "<W>"
  Bus Selector3/7 -> MATLAB Function2/7(or_w)  "<W>"
  Bus Selector2/4 -> MATLAB Function1/4(or_x)  "<X>"
  MATLAB Function8/3(transporter) -> Bus Selector4/1

== matlab function controller_stateflow_2021a/Subsystem1/MATLAB Function2 ==
  data: Time input; msgOut output Bus: SL_Bus_controller_stateflow_trajectory_msgs_JointTrajectory; msgIn input; msgPoint input; Points input; TimeFromStart input
function msgOut   = fcn(Time, msgIn, msgPoint, Points,TimeFromStart)

    msgOut = msgIn;
    if Time.Sec ~= 0

        jointNames = {'panda_joint1','panda_joint2','panda_joint3'...
            'panda_joint4','panda_joint5','panda_joint6','panda_joint7'};
        numJoints = uint32(length(jointNames));
        msgOut.JointNames_SL_Info.CurrentLength = numJoints;
        for idx = 1:numJoints
            jName = jointNames{idx};
            lenName = uint32(length(jName));
            msgOut.JointNames(idx).Data(1:lenName) = uint8(jName);
            msgOut.JointNames(idx).Data_SL_Info.CurrentLength = lenName;
        end
        
        msgOut.Points = msgPoint;
        msgOut.Points.Positions(1:7) = Points(1:7,1);
        msgOut.Points.Positions_SL_Info.CurrentLength = uint32(7);

        msgOut.Points.Velocities(1:7) = [0 ;0 ;0 ;0 ;0 ;0;0];
        msgOut.Points.Velocities_SL_Info.CurrentLength = uint32(7);
        
        msgOut.Points.Accelerations(1:7) = [0 ;0 ;0 ;0 ;0;0 ;0];
        msgOut.Points.Accelerations_SL_Info.CurrentLength = uint32(7);
        
        msgOut.Points.Effort(1:7) = [0 ;0 ;0 ;0 ;0 ;0;0];
        msgOut.Points.Effort_SL_Info.CurrentLength = uint32(7);

        msgOut.Header.Stamp.Sec = Time.Sec;
        msgOut.Header.Stamp.Nsec = Time.Nsec;
        
        msgOut.Header.Seq = uint32(0);

        msgOut.Points.TimeFromStart.Sec = TimeFromStart;
        msgOut.Points.TimeFromStart.Nsec = 0;
        msgOut.Points_SL_Info.CurrentLength = uint32(1);
    end
end

== stateflow chart controller_stateflow_2021a/Chart ==
  state wait_command
    enable = 0;
    finish_ur=0;
  state send
    enable = 1;
  state wait
    enable = 0;
  state succes
    finish_ur=1;
  (default) -> wait_command
  send -> wait
  wait_command -> send : [command == 1]
  wait -> succes : [ok == 1]
  succes -> wait_command : [command == 0]
  data: enable output; ok input; finish_ur output; command input

== matlab function controller_stateflow_2021a/Subsystem2/MATLAB Function4 ==
  data: Time input; msgOut output Bus: SL_Bus_controller_stateflow_geometry_msgs_Twist; msgIn input; sum_cntr input
function msgOut   = fcn(Time, msgIn, sum_cntr)

    msgOut = msgIn;
    if Time.Sec ~= 0
            msgOut.Linear.X = sum_cntr(1);
            msgOut.Linear.Y = sum_cntr(2);
            msgOut.Linear.Z = 0;
            msgOut.Angular.X = 0;
            msgOut.Angular.Y = 0;
            msgOut.Angular.Z = sum_cntr(3);
    end
end

== matlab function controller_stateflow_2021a/MATLAB Function ==
  data: goal input; u input; y output; tol input
function y = fcn(goal, u,tol)

    y = 0;
    
    if  u(1) <= goal(1) + tol && u(1) >= goal(1) - tol && ...
        u(2) <= goal(2) + tol && u(2) >= goal(2) - tol && ...
        u(3) <= goal(3) + tol && u(3) >= goal(3) - tol && ...
        u(4) <= goal(4) + tol && u(4) >= goal(4) - tol && ...
        u(5) <= goal(5) + tol && u(5) >= goal(5) - tol && ...
        u(6) <= goal(6) + tol && u(6) >= goal(6) - tol 
        
        y=1;
    end

== stateflow chart controller_stateflow_2021a/Chart1 ==
  state wait_command
    enable = 0;
    finish_panda=0;
  state send
    enable = 1;
  state wait
    enable = 0;
  state succes
    finish_panda=1;
  (default) -> wait_command
  wait_command -> send : [command == 1]
  send -> wait
  wait -> succes : [ok == 1]
  succes -> wait_command : [command==0]
  data: ok input; finish_panda output; command input; enable output

== matlab function controller_stateflow_2021a/MATLAB Function3 ==
  data: goal input; u input; y output; tol input
function y = fcn(goal, u,tol)

    y = 0;
    
    if  u(1) <= goal(1) + tol && u(1) >= goal(1) - tol && ...
        u(2) <= goal(2) + tol && u(2) >= goal(2) - tol && ...
        u(3) <= goal(3) + tol && u(3) >= goal(3) - tol && ...
        u(4) <= goal(4) + tol && u(4) >= goal(4) - tol && ...
        u(5) <= goal(5) + tol && u(5) >= goal(5) - tol && ...
        u(6) <= goal(6) + tol && u(6) >= goal(6) - tol && ...
        u(7) <= goal(7) + tol && u(7) >= goal(7) - tol
        y=1;
    end

== stateflow chart controller_stateflow_2021a/Chart2 ==
  state wait_command
    finish_sum=0;
  state wait
  state succes
    finish_sum=1;
  (default) -> wait_command
  wait_command -> wait : [command == 1]
  wait -> succes : [ok == 1]
  succes -> wait_command : [command==0]
  data: finish_sum output; ok input; command input

== matlab function controller_stateflow_2021a/Subsystem6/MATLAB Function1 ==
  data: pos output; x input; quat output double; y input; z input; or_x input; or_y input; or_z input; or_w input
function [pos, quat] = fcn(x,y,z,or_x,or_y,or_z,or_w)
    
    pos=[x;y;z];
    quat=[or_w;or_x;or_y;or_z];

end

== matlab function controller_stateflow_2021a/MATLAB Function5 ==
  data: goal_position input double size=[3,1]; goal_orientationZYX input double size=[3,1]; pose input; orientationZYX input; y output double size=[1,1]; tol input; sum_cntr output
function [y,sum_cntr] = fcn(goal_position, goal_orientationZYX, pose,orientationZYX,tol)

    y = 0;
    tol_or = tol+0.02;
    if  pose(1) <= goal_position(1) + tol && pose(1) >= goal_position(1) - tol && ...
        pose(2) <= goal_position(2) + tol && pose(2) >= goal_position(2) - tol && ...
        orientationZYX(1) <= goal_orientationZYX(1) + tol_or && orientationZYX(1) >= goal_orientationZYX(1) - tol_or
       
        y=1;
    end
    
    k = 0.5;
    theta = orientationZYX(1);
    e_X = k*(goal_position(1)- pose(1));
    e_Y = k*(goal_position(2)- pose(2));

    cntr_posX = e_X*cos(theta)+e_Y*sin(theta);
    cntr_posY = -e_X*sin(theta)+e_Y*cos(theta);

   

    cntr_orZ  = k*(goal_orientationZYX(1)- orientationZYX(1));
    
    sum_cntr = [cntr_posX,cntr_posY,cntr_orZ];

end

== matlab function controller_stateflow_2021a/Chart3/get_ur_pose/MATLAB Function ==
  data: Pose output; boxPos input; boxZYX input; sumPos input; sumZYX input; urState input; Weights output; initialGuess output; state input
function [Pose, Weights, initialGuess] = fcn(boxPos,boxZYX,sumPos,sumZYX,urState,state)

dimBox_x=0.38;
dimBox_y=0.18;
dimBox_z=0.14;

toSumChapa = [0;0;0.51];
toUR10e = [0.35;0.32+0.02;0.05];

boxPos_offset = [0;0;0];

velvet_length = 0.28+0.04;
velvet_height = 0.08;

base_ur_offset = [0;0;0.035];

boxtf_01 = [[eul2rotm(boxZYX', 'ZYX')],boxPos; ...
            0 0 0                               1           ];

if state == 10
    boxPos_offset = [0;-dimBox_y/2-velvet_length-0.3;-velvet_height/2-dimBox_z/2];
end

if state == 11
    boxPos_offset = [0;-dimBox_y/2-velvet_length;-velvet_height/2-dimBox_z/2];
end

if state == 12
    boxPos_offset = [0;-dimBox_y/2-velvet_length;-velvet_height/2-dimBox_z/2];
end

boxPos0 = boxtf_01*[boxPos_offset;1];

sumtf_01 = [[eul2rotm(sumZYX', 'ZYX')],sumPos; ...
            0 0 0                               1           ];
sumtoUR10etf_12 = [[eul2rotm([0,0,0], 'ZYX')],toSumChapa+toUR10e+base_ur_offset; ...
            0 0 0                               1           ];

toUR10etf = sumtf_01*sumtoUR10etf_12;


boxx = inv(toUR10etf)*[boxPos0(1:3);1];

Pose = [[eul2rotm([0,0,0], 'ZYX')],[boxx(1);boxx(2);boxx(3)]; ...
            0 0 0                               1           ];


Weights = [1,1,1,1,1,1];
initialGuess = urState(1:6,1);

end

== matlab function controller_stateflow_2021a/Subsystem6/MATLAB Function2 ==
  data: pos output; x input; quat output double; y input; z input; or_x input; or_y input; or_z input; or_w input
function [pos, quat] = fcn(x,y,z,or_x,or_y,or_z,or_w)
    
    pos=[x;y;z];
    quat=[or_w;or_x;or_y;or_z];

end

== matlab function controller_stateflow_2021a/Subsystem6/MATLAB Function8 ==
  data: box1 output Bus: SL_Bus_controller_stateflow_geometry_msgs_Pose; u input; sum_pose output Bus: SL_Bus_controller_stateflow_geometry_msgs_Pose; pose input Bus: SL_Bus_controller_stateflow_geometry_msgs_Pose; transporter output Bus: SL_Bus_controller_stateflow_geometry_msgs_Pose
function [box1,sum_pose,transporter] = fcn(u,pose)
    
    sum_pose=pose;
    idx_sum = 0;
    box1 = pose;
    idx_box1 = 0;
    transporter = pose;
    idx_tra = 0;

    linkName = uint32(length(u.Name));
    for i = 1:linkName
        link = char(u.Name(i).Data');
        link_ = deblank(link);
        if strcmp(link_,'iliad::summitxls_base_footprint')
            idx_sum = double(i);
        end
        if strcmp(link_,'box_38_18_14::link_0')
            idx_box1 = double(i);
        end
        if strcmp(link_,'transporter::link_0')
            idx_tra = double(i);
        end

    end
    
    sum_pose = u.Pose(idx_sum);
    box1 = u.Pose(idx_box1);
    transporter = u.Pose(idx_tra);

end

== matlab function controller_stateflow_2021a/Chart3/get_panda_pose/MATLAB Function ==
  data: Pose output; boxPos input; boxZYX input; sumPos input; sumZYX input; panda_state input; Weights output; initialGuess output; state input
function [Pose, Weights, initialGuess] = fcn(boxPos,boxZYX,sumPos,sumZYX,panda_state,state)

dimBox_x=0.38;
dimBox_y=0.18;
dimBox_z=0.14;

toSumChapa = [0;0;0.51];
toFranka = [0.25;-0.22;0.15];

boxPos_offset = [0;0;0];

boxtf_01 = [[eul2rotm(boxZYX', 'ZYX')],boxPos; ...
            0 0 0                               1           ];

if state == 10
    boxPos_offset = [0;dimBox_y/2-0.3;+0.3+dimBox_z/2];
end

if state == 11
    boxPos_offset = [0;dimBox_y/2;dimBox_z/2+0.05];
end

if state == 12
    boxPos_offset = [0;-dimBox_y/2-0.05;+dimBox_z/2+0.05];
end

if state == 122
    boxPos_offset = [0;+dimBox_y/2-0.06;dimBox_z/2+0.015];
end

if state == 13
    boxPos_offset = [0;0.05;0.35+dimBox_z/2];
end


% boxPos0 = boxPos+boxPos_offset;

boxPos0 = boxtf_01*[boxPos_offset;1];

sumtf_01 = [[eul2rotm(sumZYX', 'ZYX')],sumPos; ...
            0 0 0                               1           ];
sumtopandatf_12 = [[eul2rotm([0,pi/4,0], 'ZYX')],toSumChapa+toFranka; ...
            0 0 0                               1           ];

toPandatf = sumtf_01*sumtopandatf_12;

boxx = inv(toPandatf)*[boxPos0(1:3);1];


Pose = [[eul2rotm([pi,0,0], 'ZYX')],[boxx(1);boxx(2);boxx(3)]; ...
            0 0 0                               1           ];
if state == 122
    Pose = [[eul2rotm([pi,pi/8,0], 'ZYX')],[boxx(1);boxx(2);boxx(3)]; ...
            0 0 0                               1           ];
end

Weights = [1,1,1,1,1,1];


initialGuess = panda_state;

end

== stateflow chart controller_stateflow_2021a/Chart3 ==
  state ur_pos = get_ur_pose(box_pose,box_ZYX,sum_actual_pos,sum_actual_ZYX,ur_state,state) [function]
  state panda_pos = get_panda_pose(box_pos,box_ZYX,sum_actual_pos,sum_actual_ZYX,panda_state,state) [function]
  state ur_pos = get_ur_pose_tra(tra_pos,tra_ZYX,sum_actual_pos,sum_actual_ZYX,ur_state,state) [function]
  state panda_pos = get_panda_pose_track(box_pos,box_ZYX,sum_actual_pos,sum_actual_ZYX,panda_state,state) [function]
  state Initialization [group]
    state initial_state
      entry:
      fprintf("State flow started... \n");
      sum_pos = [0;0;0];
      sum_ZYX = [0;0;0];
      send_command_ur10e = 0;
      send_command_panda = 0;
      send_command_sum = 0;
      E_panda_track = 0;
      panda_durTime = 2;
      ur_durTime = 2;
      state_velvet = 0;
    state initial_pose
      entry: fprintf("Go to initial_pose \n");
      during:
      [ur_pos,ur_durTime] = set_ur_state(ur_state);
      [panda_pos,panda_durTime] = set_panda_state(panda_state);
      send_command_ur10e = 1;
      send_command_panda = 1;
      send_command_sum = 1;
    state Ready
      entry: fprintf(" initial_pose done! \n");
      send_command_ur10e = 0;
      send_command_panda = 0;
      send_command_sum = 0;
    (default) -> initial_state
    initial_state -> initial_pose : [controller_ready && link_state_ready]
    initial_pose -> Ready : [ur_finish && panda_finish && sum_finish]
  state Return home with box [group]
    state Go_back
      entry:
      send_command_sum = 0;
      display(" back ... ");
      during:
      sum_pos = [0;0;0];
      sum_ZYX = [0;0;0];
      send_command_sum = 1;
    state finish
      entry: display(" ce l'abbiamo ");
      send_command_ur10e = 0;
      send_command_panda = 0;
      send_command_sum = 0;
    Go_back -> Return.finish : [sum_finish]
  state Release box [group]
    state go_near_the_transporter
      entry:
      display(" go near the transporter ... ");
      during:
      distance_from_tra = 0.8;
      distance_xx = 0.3;
      [sum_pos,sum_ZYX] = get_sum_pose_from_tra(tra_pos,tra_ZYX,distance_from_tra,distance_xx)
      send_command_sum = 1;
    state Set_initial_ee_poses
      entry: display("set initial ee poses ");
      send_command_ur10e = 0;
      send_command_panda = 0;
      send_command_sum = 0;
      panda_durTime= 0.5;
      ur_durTime= 4;
      E_panda_track = 1;
      ur_pos = get_ur_pose_tra(tra_pos,tra_ZYX,sum_actual_pos,sum_actual_ZYX,ur_state,1);
      during:
      send_command_ur10e=1;
      panda_pos = get_panda_pose_track(box_pos,box_ZYX,sum_actual_pos,sum_actual_ZYX,panda_state,122);
    state Go_near_the_transporter
      entry:
      display(" Going near near the transporter ... ");
      send_command_ur10e = 0;
      send_command_panda = 0;
      E_panda_track = 0;
      panda_durTime = 2;
      ur_durTime = 2;
      during:
      [sum_pos,sum_ZYX] = get_sum_pose_from_tra(tra_pos,tra_ZYX,distance_from_tra,distance_xx-0.3);
      send_command_sum = 1;
    state ok
      entry: display(" gooo gooo ");
      send_command_ur10e = 0;
      send_command_panda = 0;
      send_command_sum = 0;
    state Pick_out1
      entry: display("alzo la mano");
      panda_pos = get_panda_pose(box_pos,box_ZYX,sum_actual_pos,sum_actual_ZYX,panda_state,13);
      during:
      send_command_panda = 1;
    state Pick_out2
      entry: display("lascio il box ");
      during:
      state_velvet = -1; %pick-off
    state ok1
      entry: display(" ole' ");
      send_command_ur10e = 0;
      send_command_panda = 0;
      send_command_sum = 0;
    state go_back_from_the_transporter
      entry:
      display(" go back from the transporter ... ");
      during:
      distance_from_tra = 0.8;
      distance_xx = 0.3;
      [sum_pos,sum_ZYX] = get_sum_pose_from_tra(tra_pos,tra_ZYX,distance_from_tra,distance_xx);
      send_command_sum = 1;
    go_near_the_transporter -> Release.Set_initial_ee_poses : [sum_finish && 1]
    Release.Set_initial_ee_poses -> Go_near_the_transporter : [ur_finish  && 1]
    Go_near_the_transporter -> Release.ok : [sum_finish && 1]
    Release.ok -> Pick_out1
    Pick_out1 -> Pick_out2 : [panda_finish]
    Pick_out2 -> Release.ok1 : [box_off]{state_velvet = 0;}
    Release.ok1 -> go_back_from_the_transporter
  state Pickup phase [group]
    state Go_to_Box
      entry:
      fprintf(" go near the box ... \n");
      during:
      distance_from_box = 0.8;
      distance_10 = 0.3;
      [sum_pos,sum_ZYX] = get_sum_pose_from_box(box_pos,box_ZYX,distance_from_box,distance_10);
      send_command_sum = 1;
    state Set_initial_ee_poses
      entry: fprintf("set initial ee poses ");
      send_command_ur10e = 0;
      send_command_panda = 0;
      send_command_sum = 0;
      ur_pos = get_ur_pose(box_pos,box_ZYX,sum_actual_pos,sum_actual_ZYX,ur_state,10);
      panda_pos = get_panda_pose(box_pos,box_ZYX,sum_actual_pos,sum_actual_ZYX,panda_state,10);
      during:
      send_command_ur10e=1;
      send_command_panda = 1;
    state Go_near_the_box
      entry:
      fprintf(" Going near the box ... \n");
      during:
      [sum_pos,sum_ZYX] = get_sum_pose_from_box(box_pos,box_ZYX,distance_from_box,distance_10-0.3);
      send_command_sum = 1;
    state ok
      entry: fprintf(" gooo gooo \n");
      send_command_ur10e = 0;
      send_command_panda = 0;
      send_command_sum = 0;
    state Pick_box1
      entry: fprintf("abbasso la mano \n");
      panda_pos = get_panda_pose(box_pos,box_ZYX,sum_actual_pos,sum_actual_ZYX,panda_state,11);
      during:
      send_command_panda = 1;
    state Pick_box2
      entry: fprintf("la tiro a me\n ");
      send_command_panda = 0;
      panda_pos = get_panda_pose(box_pos,box_ZYX,sum_actual_pos,sum_actual_ZYX,panda_state,12);
      during:
      send_command_panda = 1;
      state_velvet = 1; %pick-up
    state ok1
      entry: fprintf(" ole' \n");
      send_command_ur10e = 0;
      send_command_panda = 0;
      send_command_sum = 0;
    state Pick_box3
      entry: fprintf("lo teng0 \n");
      send_command_panda = 0;
      panda_pos = get_panda_pose(box_pos,box_ZYX,sum_actual_pos,sum_actual_ZYX,panda_state,122);
      during:
      send_command_panda = 1;
    state ok2
      entry: fprintf(" ole' \n");
      send_command_ur10e = 0;
      send_command_panda = 0;
      send_command_sum = 0;
    state go_back_from_the_box
      entry:
      fprintf(" go back from the box ... \n");
      distance_from_box = 0.8;
      distance_10 = 0.3;
      [sum_pos,sum_ZYX] = get_sum_pose_from_box(box_pos,box_ZYX,distance_from_box,distance_10);
      during:
      send_command_sum = 1;
    Go_to_Box -> Pickup.Set_initial_ee_poses : [sum_finish && 1]
    Pickup.Set_initial_ee_poses -> Go_near_the_box : [ur_finish && panda_finish && 1]
    Go_near_the_box -> Pickup.ok : [sum_finish && 1]
    Pickup.ok -> Pick_box1 : [1 && go]
    Pick_box1 -> Pick_box2 : [panda_finish && 1]
    Pick_box2 -> Pickup.ok1 : [panda_finish && box_on_velvet]{state_velvet = 0;}
    Pickup.ok1 -> Pick_box3
    Pick_box3 -> ok2 : [panda_finish && 1]
    ok2 -> go_back_from_the_box
  state Finish [group]
    state Return_home
      entry:
      send_command_sum = 0;
      display(" back ... ");
      during:
      sum_pos = [0;0;0];
      sum_ZYX = [0;0;0];
      [ur_pos,ur_durTime] = set_ur_state(ur_state);
      [panda_pos,panda_durTime] = set_panda_state(panda_state);
      send_command_ur10e = 1;
      send_command_panda = 1;
      send_command_sum = 1;
    state finish
      entry: display(" ce l'abbiamo ");
      send_command_ur10e = 0;
      send_command_panda = 0;
      send_command_sum = 0;
    Return_home -> Finish.finish : [ur_finish && panda_finish && sum_finish]
  state THE_END
  go_back_from_the_box -> Go_back : [sum_finish && 1]
  Return.finish -> go_near_the_transporter : [1]
  Ready -> Go_to_Box : [1]
  go_back_from_the_transporter -> Return_home : [sum_finish && 1]
  Finish.finish -> THE_END
  data: ur_stat function_input; ur_pos_ function_output; ur_durTime_ function_output; panda_pos_ function_output; panda_durTime_ function_output; panda_stat function_input; sum_pos function_output; sum_ZYX function_output; box_pos function_input; box_ZYX function_input; distance_from_box function_input; distance_10 function_input; box_pose function_input double size=[3,1]; box_ZYX function_input double size=[3,1]; sum_actual_pos function_input double size=[3,1]; sum_actual_ZYX function_input double size=[3,1]; ur_state function_input double size=[7,1]; ur_pos function_output; state function_input double size=1; box_pos function_input double size=[3,1]; box_ZYX function_input double size=[3,1]; sum_actual_pos function_input double size=[3,1]; sum_actual_ZYX function_input double size=[3,1]; panda_state function_input double size=[7,1]; panda_pos function_output; state function_input double size=1; sum_pos function_output; sum_ZYX function_output; tra_pos function_input; tra_ZYX function_input; distance_from_tra function_input; distance_xx function_input; tra_pos function_input double size=[3,1]; tra_ZYX function_input double size=[3,1]; sum_actual_pos function_input double size=[3,1]; sum_actual_ZYX function_input double size=[3,1]; ur_state function_input double size=[7,1]; ur_pos function_output; state function_input double size=1; box_pos function_input double size=[3,1]; box_ZYX function_input double size=[3,1]; sum_actual_pos function_input double size=[3,1]; sum_actual_ZYX function_input double size=[3,1]; panda_state function_input double size=[7,1]; panda_pos function_output; state function_input double size=1; sf_internal_action_state_placeholder_data local double size=1 =0; send_command_ur10e output size=1,1; controller_ready input; link_state_ready input; send_command_panda output; send_command_sum output; ur_pos output; ur_durTime output; panda_pos output; sum_pos output; panda_state input; ur_state input; panda_finish input; sum_finish input; ur_finish input; go input; box_ZYX input; sum_ZYX output; box_pos input; sum_actual_ZYX input; sum_actual_pos input; distance_10 local; distance_from_box local; box_on_velvet input; tra_ZYX input; tra_pos input; distance_from_tra local; distance_xx local; state_velvet output; E_panda_track output; panda_durTime output; box_off input
  function [ur_pos_,ur_durTime_]= set_ur_state(ur_stat):
    | function [ur_pos_,ur_durTime_]= set_ur_state(ur_stat)
    |  ur_pos_ = [0; -1.5; 2.8;-1.3; 1.57; 3.14];
    |  ur_pos_ = [       -0.6416   -5.6222+2*pi   -2.4013   -4.5429+2*pi    0.9292   -3.1416]';
    |  %ur_pos_ = [0 0 0 0 0 0]';
    |  ur_durTime_ = 3;
    | end
  function [panda_pos_,panda_durTime_] = set_panda_state(panda_stat):
    | function [panda_pos_,panda_durTime_] = set_panda_state(panda_stat)
    |  panda_pos_ = [0;-0.7853;0;-2.35619;0;1.57079;0.785398];
    |  panda_durTime_ = 3;
    | end
  function [sum_pos,sum_ZYX] = get_sum_pose_from_box(box_pos,box_ZYX,distance_from_box,distance_10):
    | function [sum_pos,sum_ZYX] = get_sum_pose_from_box(box_pos,box_ZYX,distance_from_box,distance_10)
    |     
    |     base_sum_length = 0.75; 
    | 
    |     back_from_box = box_pos - [eul2rotm(box_ZYX', 'ZYX')]*[0; distance_from_box + distance_10 + base_sum_length/2;0];
    |     
    |     sum_pos = [back_from_box(1);back_from_box(2);0];
    |     sum_ZYX = [box_ZYX(1)+pi/2;0;0];  
    | 
    | end
  function [sum_pos,sum_ZYX] = get_sum_pose_from_tra(tra_pos,tra_ZYX,distance_from_tra,distance_xx):
    | function [sum_pos,sum_ZYX] = get_sum_pose_from_tra(tra_pos,tra_ZYX,distance_from_tra,distance_xx)
    |     
    |     base_sum_length = 0.75; 
    |         
    |     traDim = [1;5.456930;0.192575];
    | 
    |     back_from_box = tra_pos + [eul2rotm(tra_ZYX', 'ZYX')]*[0; traDim(2)/2 + +0.7+distance_xx + base_sum_length/2;0];
    |     
    |     sum_pos = [back_from_box(1);back_from_box(2);0];
    |     sum_ZYX = [tra_ZYX(1)-pi/2;0;0];  
    | 
    |         
    | end

== matlab function controller_stateflow_2021a/Subsystem6/MATLAB Function10 ==
  data: pos output; x input; quat output double; y input; z input; or_x input; or_y input; or_z input; or_w input
function [pos, quat] = fcn(x,y,z,or_x,or_y,or_z,or_w)
    
    pos=[x;y;z];
    quat=[or_w;or_x;or_y;or_z];

end

== matlab function controller_stateflow_2021a/Chart3/get_ur_pose_tra/MATLAB Function ==
  data: Pose output; traPos input; traZYX input; sumPos input; sumZYX input; urState input; Weights output; initialGuess output; state input
function [Pose, Weights, initialGuess] = fcn(traPos,traZYX,sumPos,sumZYX,urState,state)

traDim = [1;5.456930;0.192575];

% back_from_box = traPos + [eul2rotm(tra_ZYX', 'ZYX')]*[0; traDim(2)/2 + +0.7+distance_xx + base_sum_length/2;0];

toSumChapa = [0;0;0.51];
toUR10e = [0.35;0.32+0.02;0.05];

traPos_offset = [0;0;0];

velvet_length = 0.28+0.04;
velvet_height = 0.08;

base_ur_offset = [0;0;0.05];

if state == 1
    traPos_offset = [eul2rotm(traZYX', 'ZYX')]*[0; traDim(2)/2 + velvet_length+0.3;-velvet_height/2+traDim(3)/2];
end
if state == 2
    traPos_offset = [eul2rotm(traZYX', 'ZYX')]*[0; traDim(2)/2 + velvet_length;-velvet_height/2+traDim(3)/2+0.1];
end


traPos0 = traPos+traPos_offset;

sumtf_01 = [[eul2rotm(sumZYX', 'ZYX')],sumPos; ...
            0 0 0                               1           ];
sumtoUR10etf_12 = [[eul2rotm([0,0,0], 'ZYX')],toSumChapa+toUR10e+base_ur_offset; ...
            0 0 0                               1           ];

toUR10etf = sumtf_01*sumtoUR10etf_12;


tra_ = inv(toUR10etf)*[traPos0;1];

Pose = [[eul2rotm([0,0,0], 'ZYX')],[tra_(1);tra_(2);tra_(3)]; ...
            0 0 0                               1           ];


Weights = [1,1,1,1,1,1];
initialGuess = urState(1:6,1);

end

== matlab function controller_stateflow_2021a/MATLAB Function1 ==
  data: u input; y output double
function y = fcn(u)
y=0;
if u.Nsec > 1e8
y=1;
end
